simulink model "sendreceiveserial"  (R2022a)
settings: Solver=VariableStepAuto  StartTime=0.0  StopTime=inf  RelTol=1e-3
undefined symbols (not defined in the file): LF
libraries: simulink x3, instrumentseriallib x3
settings Model: Creator=ashal  LastModifiedBy=ashal
settings SFSimCC: SimTargetLang=C++

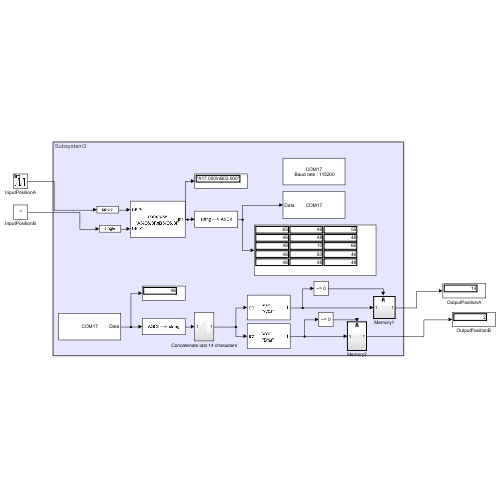
[thumbnail: Simulink's stored preview of the top-level diagram]
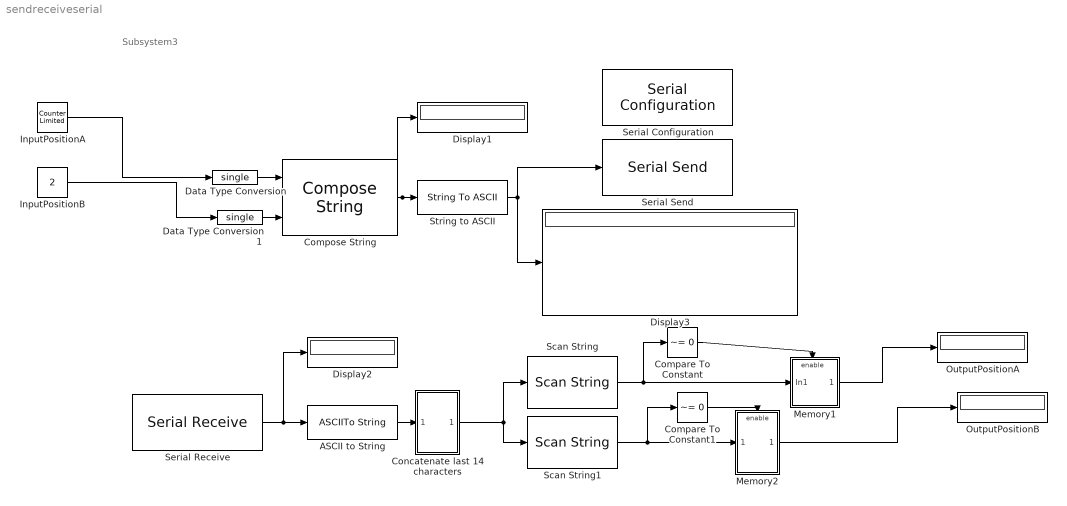
== system sendreceiveserial ==
  note: Subsystem3
  ASCII to String : ASCIIToString
  Compare To Constant : simulink/Logic and Bit Operations/Compare To Constant  relop=~=  const=0  OutDataTypeStr=boolean
  Compare To Constant1 : simulink/Logic and Bit Operations/Compare To Constant  relop=~=  const=0  OutDataTypeStr=boolean
  Compose String : ComposeString  Format="\"A%06.3f\\nB%06.3f\""
  Concatenate last 14 characters : Subsystem
  Data Type Conversion : DataTypeConversion  OutDataTypeStr=single  SaturateOnIntegerOverflow=off  RndMeth=Floor  LockScale=on
  Data Type Conversion1 : DataTypeConversion  OutDataTypeStr=single  SaturateOnIntegerOverflow=off  RndMeth=Floor  LockScale=on
  Display1 : Display
  Display2 : Display
  Display3 : Display
  InputPositionA : simulink/Sources/Counter Limited  uplimit=40  tsamp=-1
  InputPositionB : Constant  Value=2  OutDataTypeStr=single
  Memory1 : Subsystem
  Memory2 : Subsystem
  OutputPositionA : Display
  OutputPositionB : Display
  Scan String : ScanString  Format="\"A%f\""
  Scan String1 : ScanString  Format="\"B%f\""
  Serial Configuration : instrumentseriallib/Serial Configuration  Priority=-200000  PortSel=COM17  Port=COM17  ComPort=COM17  BaudRate=115200  DataBits=8  Parity=none  StopBits=1  ByteOrder=little-endian  FlowControl=none  Timeout=10  SimulateUsing=Interpreted execution  BlockInModel=on  aMode=1
      settings: SourceProductBaseCode=OT,IC,MT
  Serial Receive : instrumentseriallib/Serial Receive  Priority=1  PortSel=COM17  Port=COM17  ComPort=COM17  DataType=uint8  SaveDataType=uint8  ToggleHeader=off  Header=[]  ToggleTerminator=on  Terminator=<none>  CustomTerminator=[]  InputFormat=Column major  ToggleDataSize=on  DataSize=ones(1, 128);  EnableBlockingMode=on  ActionDataUnavailable=Output last received value  ActionWhenDataUnavailable=Output last received value  CustomValue=0  SampleTime=0.01  SimulateUsing=Interpreted execution  BlockInModel=on  aMode=1
      settings: SourceProductBaseCode=OT,IC,MT
  Serial Send : instrumentseriallib/Serial Send  Priority=1  PortSel=COM17  Port=COM17  ComPort=COM17  Header=[]  Terminator=LF ('\n')  CustomTerminator=[]  EnableBlockingMode=on  SimulateUsing=Interpreted execution  BlockInModel=on  aMode=1
      settings: SourceProductBaseCode=OT,IC,MT
  String to ASCII : StringToASCII  OutputVectorSize=15
  wires:
  Memory1/1(Out1) -> OutputPositionA/1
  Memory2/1(Out1) -> OutputPositionB/1
  InputPositionB/1 -> Data Type Conversion1/1
  InputPositionA/1 -> Data Type Conversion/1
  Serial Receive/1 -> ASCII to String/1, Display2/1
  Compare To Constant/1 -> Memory1/Enable
  Compose String/1 -> Display1/1, String to ASCII/1
  Concatenate last 14 characters/1(Out1) -> Scan String1/1, Scan String/1
  Data Type Conversion/1 -> Compose String/1
  String to ASCII/1 -> Serial Send/1, Display3/1
  Data Type Conversion1/1 -> Compose String/2
  Scan String/1 -> Memory1/1(In1), Compare To Constant/1
  ASCII to String/1 -> Concatenate last 14 characters/1(In1)
  Compare To Constant1/1 -> Memory2/Enable
  Scan String1/1 -> Compare To Constant1/1, Memory2/1(In1)

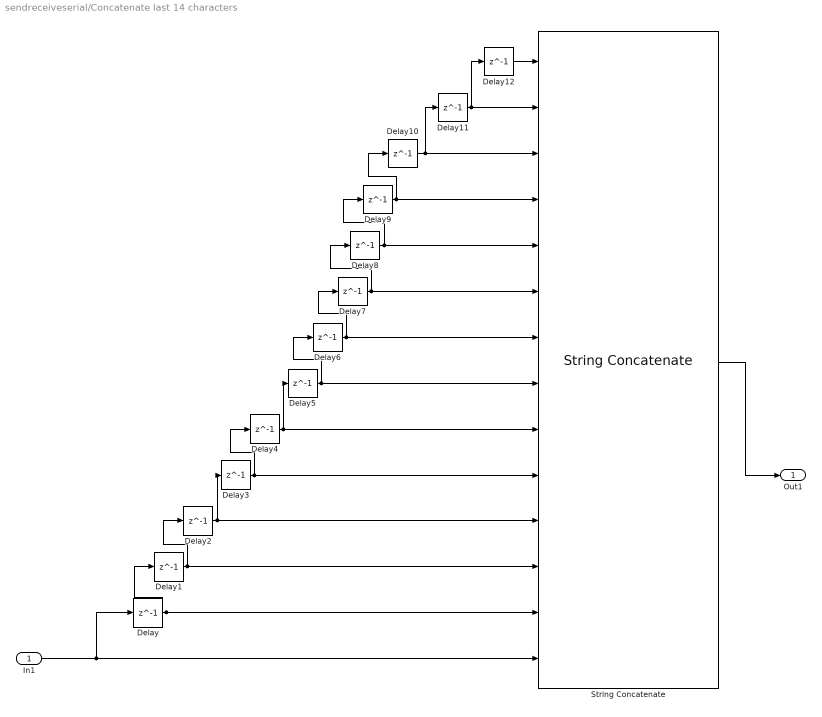
== system sendreceiveserial/Concatenate last 14 characters ==
  In1 : Inport
  Delay{,1..12} (13 alike) : Delay  DelayLength=1
  String Concatenate : StringConcatenate  Inputs=14
  Out1 : Outport
  wires:
  String Concatenate/1 -> Out1/1
  In1/1 -> String Concatenate/14, Delay/1
  Delay/1 -> Delay1/1, String Concatenate/13
  Delay1/1 -> Delay2/1, String Concatenate/12
  Delay2/1 -> Delay3/1, String Concatenate/11
  Delay3/1 -> Delay4/1, String Concatenate/10
  Delay4/1 -> Delay5/1, String Concatenate/9
  Delay5/1 -> Delay6/1, String Concatenate/8
  Delay6/1 -> Delay7/1, String Concatenate/7
  Delay7/1 -> Delay8/1, String Concatenate/6
  Delay8/1 -> Delay9/1, String Concatenate/5
  Delay9/1 -> Delay10/1, String Concatenate/4
  Delay10/1 -> Delay11/1, String Concatenate/3
  Delay11/1 -> Delay12/1, String Concatenate/2
  Delay12/1 -> String Concatenate/1

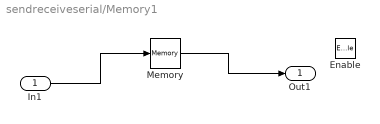
== system sendreceiveserial/Memory1 ==
  In1 : Inport
  Enable : EnablePort
  Memory : Memory
  Out1 : Outport
  wires:
  In1/1 -> Memory/1
  Memory/1 -> Out1/1

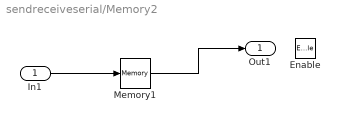
== system sendreceiveserial/Memory2 ==
  In1 : Inport
  Enable : EnablePort
  Memory1 : Memory
  Out1 : Outport
  wires:
  In1/1 -> Memory1/1
  Memory1/1 -> Out1/1
